simulink model "d_009_classicalGen_nonunidamp"  (Simulink 9.2)
settings: Solver=ode3  StartTime=0.0  StopTime=10.0  FixedStep=1e-4  RelTol=1e-3  EnableMultiTasking=on
libraries: fm_lib x2
settings Model: Creator=fmilano  LastModifiedBy=sl48876  ExtModeAutoUpdateStatusClock=off
settings OptimizationCC: BooleanDataType=off  InitFltsAndDblsToZero=on
settings DebuggingCC: SaveWithParameterizedLinksMsg=none  SignalResolutionControl=TryResolveAllWithWarning  MultiTaskDSMMsg=warning  MultiTaskCondExecSysMsg=none  FcnCallInpInsideContextMsg=error  StateNameClashWarn=none
settings HardwareCC: TargetUnknown=on
settings GRTTargetCC: TargetFcnLib=ansi_tfl_tmw.mat  CodeReplacementLibrary=ANSI_C  CompOptLevelCompliant=off  CPPClassGenCompliant=off
settings ConfigComp: CovSFcnEnable=off

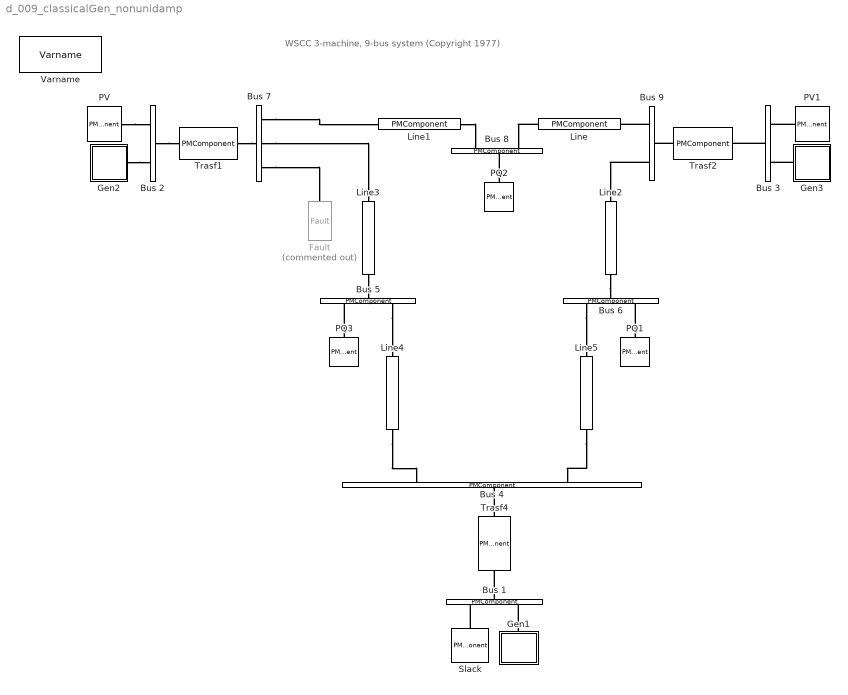
== system d_009_classicalGen_nonunidamp ==
  note: WSCC 3-machine, 9-bus system (Copyright 1977)
  Bus 1 : PMComponent  Tag=PSATblock  Description=Connection  PhysicalDomain=psatdomain  LeftPortType=p1  RightPortType=p1  LConnTagsString=__newl0|__newl1  RConnTagsString=__newr0  mask(Bus){in=2, out=1, p2q=16.5, p3_4q=[1.00   0.00], p5q=4, p6q=1}
      mask prompts: in "Number of inputs:"; out "Number of outputs:"; p2q "Voltage Rating [kV]"; p3_4q "Voltage initial guess [p.u.  rad]"; p5q "Area number"; p6q "Region number"
      mask help: Bus block.
      mask init:
      | fm_inout
      mask Callback p5q: fm_block
      mask Display: plot([0 1 1 0 0],[0 0 1 1 0])
  Bus 2 : PMComponent  Tag=PSATblock  Description=Connection  PhysicalDomain=psatdomain  LeftPortType=p1  RightPortType=p1  LConnTagsString=__newl0|__newl1  RConnTagsString=__newr0  mask(Bus){in=2, out=1, p2q=18, p3_4q=[1.00   0.00], p5q=5, p6q=1}
      mask prompts: in "Number of inputs:"; out "Number of outputs:"; p2q "Voltage Rating [kV]"; p3_4q "Voltage initial guess [p.u.  rad]"; p5q "Area number"; p6q "Region number"
      mask help: Bus block.
      mask init:
      | fm_inout
      mask Callback p5q: fm_block
      mask Display: plot([0 1 1 0 0],[0 0 1 1 0])
  Bus 3 : PMComponent  Tag=PSATblock  Description=Connection  PhysicalDomain=psatdomain  LeftPortType=p1  RightPortType=p1  LConnTagsString=__newl0|__newl1  RConnTagsString=__newr0  mask(Bus){in=2, out=1, p2q=13.8, p3_4q=[1.00   0.00], p5q=3, p6q=1}
      mask prompts: in "Number of inputs:"; out "Number of outputs:"; p2q "Voltage Rating [kV]"; p3_4q "Voltage initial guess [p.u.  rad]"; p5q "Area number"; p6q "Region number"
      mask help: Bus block.
      mask init:
      | fm_inout
      mask Callback p5q: fm_block
      mask Display: plot([0 1 1 0 0],[0 0 1 1 0])
  Bus 4 : PMComponent  Tag=PSATblock  Description=Connection  PhysicalDomain=psatdomain  LeftPortType=p1  RightPortType=p1  LConnTagsString=__newl0|__newl1  RConnTagsString=__newr0  mask(Bus){in=2, out=1, p2q=230, p3_4q=[1.00   0.00], p5q=2, p6q=1}
      mask prompts: in "Number of inputs:"; out "Number of outputs:"; p2q "Voltage Rating [kV]"; p3_4q "Voltage initial guess [p.u.  rad]"; p5q "Area number"; p6q "Region number"
      mask help: Bus block.
      mask init:
      | fm_inout
      mask Callback p5q: fm_block
      mask Display: plot([0 1 1 0 0],[0 0 1 1 0])
  Bus 5 : PMComponent  Tag=PSATblock  Description=Connection  PhysicalDomain=psatdomain  LeftPortType=p1  RightPortType=p1  LConnTagsString=__newl0  RConnTagsString=__newr0|__newr1  mask(Bus){in=1, out=2, p2q=230, p3_4q=[1.00   0.00], p5q=2, p6q=1}
      mask prompts: in "Number of inputs:"; out "Number of outputs:"; p2q "Voltage Rating [kV]"; p3_4q "Voltage initial guess [p.u.  rad]"; p5q "Area number"; p6q "Region number"
      mask help: Bus block.
      mask init:
      | fm_inout
      mask Callback p5q: fm_block
      mask Display: plot([0 1 1 0 0],[0 0 1 1 0])
  Bus 6 : PMComponent  Tag=PSATblock  Description=Connection  PhysicalDomain=psatdomain  LeftPortType=p1  RightPortType=p1  LConnTagsString=__newl0  RConnTagsString=__newr0|__newr1  mask(Bus){in=1, out=2, p2q=230, p3_4q=[1.00   0.00], p5q=2, p6q=1}
      mask prompts: in "Number of inputs:"; out "Number of outputs:"; p2q "Voltage Rating [kV]"; p3_4q "Voltage initial guess [p.u.  rad]"; p5q "Area number"; p6q "Region number"
      mask help: Bus block.
      mask init:
      | fm_inout
      mask Callback p5q: fm_block
      mask Display: plot([0 1 1 0 0],[0 0 1 1 0])
  Bus 7 : PMComponent  Tag=PSATblock  Description=Connection  PhysicalDomain=psatdomain  LeftPortType=p1  RightPortType=p1  LConnTagsString=__newl0  RConnTagsString=__newr0|__newr1|__newr2  mask(Bus){in=1, out=3, p2q=230, p3_4q=[1.00   0.00], p5q=2, p6q=1}
      mask prompts: in "Number of inputs:"; out "Number of outputs:"; p2q "Voltage Rating [kV]"; p3_4q "Voltage initial guess [p.u.  rad]"; p5q "Area number"; p6q "Region number"
      mask help: Bus block.
      mask init:
      | fm_inout
      mask Callback p5q: fm_block
      mask Display: plot([0 1 1 0 0],[0 0 1 1 0])
  Bus 8 : PMComponent  Tag=PSATblock  Description=Connection  PhysicalDomain=psatdomain  LeftPortType=p1  RightPortType=p1  LConnTagsString=__newl0|__newl1  RConnTagsString=__newr0  mask(Bus){in=2, out=1, p2q=230, p3_4q=[1.00   0.00], p5q=2, p6q=1}
      mask prompts: in "Number of inputs:"; out "Number of outputs:"; p2q "Voltage Rating [kV]"; p3_4q "Voltage initial guess [p.u.  rad]"; p5q "Area number"; p6q "Region number"
      mask help: Bus block.
      mask init:
      | fm_inout
      mask Callback p5q: fm_block
      mask Display: plot([0 1 1 0 0],[0 0 1 1 0])
  Bus 9 : PMComponent  Tag=PSATblock  Description=Connection  PhysicalDomain=psatdomain  LeftPortType=p1  RightPortType=p1  LConnTagsString=__newl0  RConnTagsString=__newr0|__newr1  mask(Bus){in=1, out=2, p2q=230, p3_4q=[1.00   0.00], p5q=2, p6q=1}
      mask prompts: in "Number of inputs:"; out "Number of outputs:"; p2q "Voltage Rating [kV]"; p3_4q "Voltage initial guess [p.u.  rad]"; p5q "Area number"; p6q "Region number"
      mask help: Bus block.
      mask init:
      | fm_inout
      mask Callback p5q: fm_block
      mask Display: plot([0 1 1 0 0],[0 0 1 1 0])
  Fault : fm_lib/Faults &  Breakers/Fault  Tag=PSATblock  Description=Faults & Breakers  Commented=on  LConnTagsString=__newl0  p2_3_4q="[100  400  60]"  p5q=1.00  p6q=1.0025  p7q=1e-5  p8q=1e-3
  Gen1 : Subsystem  Tag=PSATblock  Description=Machines  mask(Syn){p2_3_4q=[100  16.5   60], p5q=2, p7_6q=[0.00  0.00], p8_9_10q=[0.1460  0.0608  0.0000], p11_12q=[8.96  0.00], p13_14_15q=[0.0969  0.0969  0.0000], p16_17q=[0.310  0.0000], p18_19q=[2*23.64  0.1*47.28], p20_21q=[0.00  0.00], p22_23q=[1.00  1.00], p24q=0.002, p25_26q=[0 0], in=0, p27q=1, p28q=on}
      mask prompts: p2_3_4q "Power, voltage and frequency ratings [MVA, kV, Hz]"; p5q "Machine Dynamic Order"; p7_6q "resistance ra and leakage reactance xl [p.u. p.u.]"; p8_9_10q "d-axis reactances Xd, X'd X"d [p.u.,p.u.,p.u.]"; p11_12q "d-axis open circuit time constants T'd0 and T"d0 [s, s]"; p13_14_15q "q-axis reactances Xq, X'q, X"q [p.u.  p.u.  p.u.]"; p16_17q "q-axis open circuit time constants T'q0 and T"q0 [s s]"; p18_19q "Inertia (M = 2H) and Damping [s, p.u.]"; p20_21q "Speed and active power additional signals Kw and Kp [p.u., p.u.]"; p22_23q "Percentage of active and reactive powers at bus [p.u. p.u.]"; p24q "d-axis additional circuit leakage time constant Taa [s]"; p25_26q "Saturation coefficients S(1.0) and S(1.2)"; in "Number of input signals"; p27q "COI number"; p28q "Connected"
      mask help: This block defines a fourth order synchronous machine.
      mask init:
      | fm_inout
      | [x,y] = fm_draw('circle');
      | [xg,yg] = fm_draw('G');
      | [xs,ys] = fm_draw('sinus');
      mask TypeOptions p5q: 8 | 6 | 5.3 | 5.2 | 5.1 | 4 | 3 | 2
      mask Callback p5q: fm_block
      mask TypeOptions in: 0 | 1 | 2
      mask Callback p28q: fm_block
      mask Display:
      | plot(x+1.4,y,0.12*xs+1,0.15*ys-0.6)
      | color('blue')
      | plot(1.4+0.45*xg,0.3+0.45*yg)
  Gen2 : Subsystem  Tag=PSATblock  Description=Machines  mask(Syn){p2_3_4q=[100  18   60], p5q=2, p7_6q=[0.00  0.00], p8_9_10q=[0.8958  0.1198  0.0000], p11_12q=[6.00  0.00], p13_14_15q=[0.8645  0.1969  0.0000], p16_17q=[0.5350  0.0000], p18_19q=[12.80  0.2*12.80], p20_21q=[0.00  0.00], p22_23q=[1.00  1.00], p24q=0.002, p25_26q=[0 0], in=0, p27q=1, p28q=on}
      mask prompts: p2_3_4q "Power, voltage and frequency ratings [MVA, kV, Hz]"; p5q "Machine Dynamic Order"; p7_6q "resistance ra and leakage reactance xl [p.u. p.u.]"; p8_9_10q "d-axis reactances Xd, X'd X"d [p.u.,p.u.,p.u.]"; p11_12q "d-axis open circuit time constants T'd0 and T"d0 [s, s]"; p13_14_15q "q-axis reactances Xq, X'q, X"q [p.u.  p.u.  p.u.]"; p16_17q "q-axis open circuit time constants T'q0 and T"q0 [s s]"; p18_19q "Inertia (M = 2H) and Damping [s, p.u.]"; p20_21q "Speed and active power additional signals Kw and Kp [p.u., p.u.]"; p22_23q "Percentage of active and reactive powers at bus [p.u. p.u.]"; p24q "d-axis additional circuit leakage time constant Taa [s]"; p25_26q "Saturation coefficients S(1.0) and S(1.2)"; in "Number of input signals"; p27q "COI number"; p28q "Connected"
      mask help: This block defines a fourth order synchronous machine.
      mask init:
      | fm_inout
      | [x,y] = fm_draw('circle');
      | [xg,yg] = fm_draw('G');
      | [xs,ys] = fm_draw('sinus');
      mask TypeOptions p5q: 8 | 6 | 5.3 | 5.2 | 5.1 | 4 | 3 | 2
      mask Callback p5q: fm_block
      mask TypeOptions in: 0 | 1 | 2
      mask Callback p28q: fm_block
      mask Display:
      | plot(x+1.4,y,0.12*xs+1,0.15*ys-0.6)
      | color('blue')
      | plot(1.4+0.45*xg,0.3+0.45*yg)
  Gen3 : Subsystem  Tag=PSATblock  Description=Machines  mask(Syn){p2_3_4q=[100  13.8   60], p5q=2, p7_6q=[0.00  0.00], p8_9_10q=[1.3125  0.1813  0.0000], p11_12q=[5.89  0.00], p13_14_15q=[1.2578  0.2500  0.0000], p16_17q=[0.600  0.0000], p18_19q=[6.02  0.3*6.02], p20_21q=[0.00  0.00], p22_23q=[1.00  1.00], p24q=0.002, p25_26q=[0 0], in=0, p27q=1, p28q=on}
      mask prompts: p2_3_4q "Power, voltage and frequency ratings [MVA, kV, Hz]"; p5q "Machine Dynamic Order"; p7_6q "resistance ra and leakage reactance xl [p.u. p.u.]"; p8_9_10q "d-axis reactances Xd, X'd X"d [p.u.,p.u.,p.u.]"; p11_12q "d-axis open circuit time constants T'd0 and T"d0 [s, s]"; p13_14_15q "q-axis reactances Xq, X'q, X"q [p.u.  p.u.  p.u.]"; p16_17q "q-axis open circuit time constants T'q0 and T"q0 [s s]"; p18_19q "Inertia (M = 2H) and Damping [s, p.u.]"; p20_21q "Speed and active power additional signals Kw and Kp [p.u., p.u.]"; p22_23q "Percentage of active and reactive powers at bus [p.u. p.u.]"; p24q "d-axis additional circuit leakage time constant Taa [s]"; p25_26q "Saturation coefficients S(1.0) and S(1.2)"; in "Number of input signals"; p27q "COI number"; p28q "Connected"
      mask help: This block defines a fourth order synchronous machine.
      mask init:
      | fm_inout
      | [x,y] = fm_draw('circle');
      | [xg,yg] = fm_draw('G');
      | [xs,ys] = fm_draw('sinus');
      mask TypeOptions p5q: 8 | 6 | 5.3 | 5.2 | 5.1 | 4 | 3 | 2
      mask Callback p5q: fm_block
      mask TypeOptions in: 0 | 1 | 2
      mask Callback p28q: fm_block
      mask Display:
      | plot(x+1.4,y,0.12*xs+1,0.15*ys-0.6)
      | color('blue')
      | plot(1.4+0.45*xg,0.3+0.45*yg)
  Line : PMComponent  Tag=PSATblock  Description=Power Flow  PhysicalDomain=psatdomain  LeftPortType=p1  RightPortType=p1  LConnTagsString=__newl0  RConnTagsString=__newr0  mask(Line){p3_4_5q=[100  230  60], p6q=0, p8q=0.0119, p9q=0.1008, p10q=0.1045*2, p13_14_15q=[0.0  0.0  0.0], p16q=on}
      mask prompts: p3_4_5q "Power, Voltage and Frequency Ratings [MVA, kV, Hz]"; p6q "Length of line [km] (0 for p.u. parameters)"; p8q "Resistance [p.u. (Ohms/km)]"; p9q "Reactance [p.u. (H/km)]"; p10q "Susceptance [p.u. (F/km)]"; p13_14_15q "Imax, Pmax and Smax [p.u., p.u., p.u.]"; p16q "Connected"
      mask help: This block defines a pi model for a tree phase line.
      mask init:
      | [xp,yp] = fm_draw('pi');
      mask Callback p16q: fm_block
      mask Display:
      | plot([-1  1  1 -1 -1],[-0.2 -0.2 0.2 0.2 -0.2])
      | color('blue')
      | plot(0.35*xp,0.2*yp)
  Line1 : PMComponent  Tag=PSATblock  Description=Power Flow  PhysicalDomain=psatdomain  LeftPortType=p1  RightPortType=p1  LConnTagsString=__newl0  RConnTagsString=__newr0  mask(Line){p3_4_5q=[100  230  60], p6q=0, p8q=0.0085, p9q=0.072*5, p10q=0.0745*2, p13_14_15q=[0.0  0.0  0.0], p16q=on}
      mask prompts: p3_4_5q "Power, Voltage and Frequency Ratings [MVA, kV, Hz]"; p6q "Length of line [km] (0 for p.u. parameters)"; p8q "Resistance [p.u. (Ohms/km)]"; p9q "Reactance [p.u. (H/km)]"; p10q "Susceptance [p.u. (F/km)]"; p13_14_15q "Imax, Pmax and Smax [p.u., p.u., p.u.]"; p16q "Connected"
      mask help: This block defines a pi model for a tree phase line.
      mask init:
      | [xp,yp] = fm_draw('pi');
      mask Callback p16q: fm_block
      mask Display:
      | plot([-1  1  1 -1 -1],[-0.2 -0.2 0.2 0.2 -0.2])
      | color('blue')
      | plot(0.35*xp,0.2*yp)
  Line2 : PMComponent  Tag=PSATblock  Description=Power Flow  PhysicalDomain=psatdomain  LeftPortType=p1  RightPortType=p1  LConnTagsString=__newl0  RConnTagsString=__newr0  mask(Line){p3_4_5q=[100  230  60], p6q=0, p8q=0.039, p9q=0.170*5, p10q=0.179*2, p13_14_15q=[0.0  0.0  0.0], p16q=on}
      mask prompts: p3_4_5q "Power, Voltage and Frequency Ratings [MVA, kV, Hz]"; p6q "Length of line [km] (0 for p.u. parameters)"; p8q "Resistance [p.u. (Ohms/km)]"; p9q "Reactance [p.u. (H/km)]"; p10q "Susceptance [p.u. (F/km)]"; p13_14_15q "Imax, Pmax and Smax [p.u., p.u., p.u.]"; p16q "Connected"
      mask help: This block defines a pi model for a tree phase line.
      mask init:
      | [xp,yp] = fm_draw('pi');
      mask Callback p16q: fm_block
      mask Display:
      | plot([-1  1  1 -1 -1],[-0.2 -0.2 0.2 0.2 -0.2])
      | color('blue')
      | plot(0.35*xp,0.2*yp)
  Line3 : PMComponent  Tag=PSATblock  Description=Power Flow  PhysicalDomain=psatdomain  LeftPortType=p1  RightPortType=p1  LConnTagsString=__newl0  RConnTagsString=__newr0  mask(Line){p3_4_5q=[100  230  60], p6q=0, p8q=0.032, p9q=0.161*5, p10q=0.153*2, p13_14_15q=[0.0  0.0  0.0], p16q=on}
      mask prompts: p3_4_5q "Power, Voltage and Frequency Ratings [MVA, kV, Hz]"; p6q "Length of line [km] (0 for p.u. parameters)"; p8q "Resistance [p.u. (Ohms/km)]"; p9q "Reactance [p.u. (H/km)]"; p10q "Susceptance [p.u. (F/km)]"; p13_14_15q "Imax, Pmax and Smax [p.u., p.u., p.u.]"; p16q "Connected"
      mask help: This block defines a pi model for a tree phase line.
      mask init:
      | [xp,yp] = fm_draw('pi');
      mask Callback p16q: fm_block
      mask Display:
      | plot([-1  1  1 -1 -1],[-0.2 -0.2 0.2 0.2 -0.2])
      | color('blue')
      | plot(0.35*xp,0.2*yp)
  Line4 : PMComponent  Tag=PSATblock  Description=Power Flow  PhysicalDomain=psatdomain  LeftPortType=p1  RightPortType=p1  LConnTagsString=__newl0  RConnTagsString=__newr0  mask(Line){p3_4_5q=[100  230  60], p6q=0, p8q=0.01, p9q=0.085, p10q=0.088*2, p13_14_15q=[0.0  0.0  0.0], p16q=on}
      mask prompts: p3_4_5q "Power, Voltage and Frequency Ratings [MVA, kV, Hz]"; p6q "Length of line [km] (0 for p.u. parameters)"; p8q "Resistance [p.u. (Ohms/km)]"; p9q "Reactance [p.u. (H/km)]"; p10q "Susceptance [p.u. (F/km)]"; p13_14_15q "Imax, Pmax and Smax [p.u., p.u., p.u.]"; p16q "Connected"
      mask help: This block defines a pi model for a tree phase line.
      mask init:
      | [xp,yp] = fm_draw('pi');
      mask Callback p16q: fm_block
      mask Display:
      | plot([-1  1  1 -1 -1],[-0.2 -0.2 0.2 0.2 -0.2])
      | color('blue')
      | plot(0.35*xp,0.2*yp)
  Line5 : PMComponent  Tag=PSATblock  Description=Power Flow  PhysicalDomain=psatdomain  LeftPortType=p1  RightPortType=p1  LConnTagsString=__newl0  RConnTagsString=__newr0  mask(Line){p3_4_5q=[100  230  60], p6q=0, p8q=0.017, p9q=0.092, p10q=0.079*2, p13_14_15q=[0.0  0.0  0.0], p16q=on}
      mask prompts: p3_4_5q "Power, Voltage and Frequency Ratings [MVA, kV, Hz]"; p6q "Length of line [km] (0 for p.u. parameters)"; p8q "Resistance [p.u. (Ohms/km)]"; p9q "Reactance [p.u. (H/km)]"; p10q "Susceptance [p.u. (F/km)]"; p13_14_15q "Imax, Pmax and Smax [p.u., p.u., p.u.]"; p16q "Connected"
      mask help: This block defines a pi model for a tree phase line.
      mask init:
      | [xp,yp] = fm_draw('pi');
      mask Callback p16q: fm_block
      mask Display:
      | plot([-1  1  1 -1 -1],[-0.2 -0.2 0.2 0.2 -0.2])
      | color('blue')
      | plot(0.35*xp,0.2*yp)
  PQ1 : PMComponent  Tag=PSATblock  Description=Power Flow  PhysicalDomain=psatdomain  LeftPortType=p1  RightPortType=p1  LConnTagsString=__newl0  mask(PQ){p2_3q=[100  230], p4_5q=[0.90  0.30], p6_7q=[1.2  0.8], p8q=off, p9q=on}
      mask prompts: p2_3q "Power and Voltage Ratings [MVA, kV]"; p4_5q "Active and Reactive Powers [p.u.  p.u.]"; p6_7q "Maximum and Minimum Allowable Voltage [p.u.   p.u.]"; p8q "Allow conversion to impendance for min & max voltage"; p9q "Connected"
      mask help:
      | This block defines a constant power load:
      |
      | P = Pcost.
      | Q = Qcost.
      mask Callback p8q: fm_block
      mask Callback p9q: fm_block
      mask Display: plot([1 -0.5 -0.5 1],[0 0.866 -0.866 0])
  PQ2 : PMComponent  Tag=PSATblock  Description=Power Flow  PhysicalDomain=psatdomain  LeftPortType=p1  RightPortType=p1  LConnTagsString=__newl0  mask(PQ){p2_3q=[100  230], p4_5q=[1.00  0.35], p6_7q=[1.2  0.8], p8q=off, p9q=on}
      mask prompts: p2_3q "Power and Voltage Ratings [MVA, kV]"; p4_5q "Active and Reactive Powers [p.u.  p.u.]"; p6_7q "Maximum and Minimum Allowable Voltage [p.u.   p.u.]"; p8q "Allow conversion to impendance for min & max voltage"; p9q "Connected"
      mask help:
      | This block defines a constant power load:
      |
      | P = Pcost.
      | Q = Qcost.
      mask Callback p8q: fm_block
      mask Callback p9q: fm_block
      mask Display: plot([1 -0.5 -0.5 1],[0 0.866 -0.866 0])
  PQ3 : PMComponent  Tag=PSATblock  Description=Power Flow  PhysicalDomain=psatdomain  LeftPortType=p1  RightPortType=p1  LConnTagsString=__newl0  mask(PQ){p2_3q=[100  230], p4_5q=[1.25  0.50], p6_7q=[1.2  0.8], p8q=off, p9q=on}
      mask prompts: p2_3q "Power and Voltage Ratings [MVA, kV]"; p4_5q "Active and Reactive Powers [p.u.  p.u.]"; p6_7q "Maximum and Minimum Allowable Voltage [p.u.   p.u.]"; p8q "Allow conversion to impendance for min & max voltage"; p9q "Connected"
      mask help:
      | This block defines a constant power load:
      |
      | P = Pcost.
      | Q = Qcost.
      mask Callback p8q: fm_block
      mask Callback p9q: fm_block
      mask Display: plot([1 -0.5 -0.5 1],[0 0.866 -0.866 0])
  PV : PMComponent  Tag=PSATblock  Description=Power Flow  PhysicalDomain=psatdomain  LeftPortType=p1  RightPortType=p1  RConnTagsString=__newr0  mask(PV){p2_3q=[100  18], p4q=1.63, p5q=1.025, p6_7q=[99 -99], p8_9q=[1.1  0.9], p10q=1, p11q=on}
      mask prompts: p2_3q "Power and Voltage Ratings [MVA, kV]"; p4q "Active Power [p.u.]"; p5q "Voltage Magnitude [p.u.]"; p6_7q "Qmax and Qmin [p.u.  p.u.]"; p8_9q "Vmax and Vmin [p.u.  p.u.]"; p10q "Loss Participation Factor"; p11q "Connected"
      mask help:
      | This block defines a PV bus for load flow studies:
      |
      | P = Pcost.
      | V = Vdes.
      mask init:
      | [x,y] = fm_draw('circle');
      | [xp,yp] = fm_draw('P');
      mask Callback p11q: fm_block
      mask Display:
      | plot(x,y)
      | color('blue')
      | plot(0.3*xp-0.35,0.6*yp,[0.1 0.3 0.5],[0.3 -0.3 0.3])
  PV1 : PMComponent  Tag=PSATblock  Description=Power Flow  PhysicalDomain=psatdomain  LeftPortType=p1  RightPortType=p1  RConnTagsString=__newr0  mask(PV){p2_3q=[100  13.8], p4q=0.85, p5q=1.025, p6_7q=[99  -99], p8_9q=[1.1  0.9], p10q=1, p11q=on}
      mask prompts: p2_3q "Power and Voltage Ratings [MVA, kV]"; p4q "Active Power [p.u.]"; p5q "Voltage Magnitude [p.u.]"; p6_7q "Qmax and Qmin [p.u.  p.u.]"; p8_9q "Vmax and Vmin [p.u.  p.u.]"; p10q "Loss Participation Factor"; p11q "Connected"
      mask help:
      | This block defines a PV bus for load flow studies:
      |
      | P = Pcost.
      | V = Vdes.
      mask init:
      | [x,y] = fm_draw('circle');
      | [xp,yp] = fm_draw('P');
      mask Callback p11q: fm_block
      mask Display:
      | plot(x,y)
      | color('blue')
      | plot(0.3*xp-0.35,0.6*yp,[0.1 0.3 0.5],[0.3 -0.3 0.3])
  Slack : PMComponent  Tag=PSATblock  Description=Power Flow  PhysicalDomain=psatdomain  LeftPortType=p1  RightPortType=p1  RConnTagsString=__newr0  mask(SW){p2_3q=[100  16.5], p4q=1.04, p5q=0.00, p6_7q=[99 -99], p8_9q=[1.1  0.9], p10q=0.80, p11q=1, p12q=on, p13q=on}
      mask prompts: p2_3q "Power and Voltage Ratings [MVA, kV]"; p4q "Voltage Magnitude [p.u.]"; p5q "Reference Phase Angle [rad]"; p6_7q "Qmax and Qmin [p.u.  p.u.]"; p8_9q "Vmax and Vmin  [p.u.  p.u.]"; p10q "Active Power Guess [p.u.]"; p11q "Loss Participation Factor"; p12q "Reference bus"; p13q "Connected"
      mask help:
      | This block defines a V-theta bus:
      |
      | V = V_des
      | theta = theta_des
      mask init:
      | [x,y] = fm_draw('circle');
      | [xt,yt] = fm_draw('theta');
      mask Callback p12q: fm_block
      mask Callback p13q: fm_block
      mask Display: plot([0 1 1 0 0],[0 0 1 1 0]), color('blue'), plot([0 1],[0 1],[0 1],[1 0],[0.5 1 0.5 0 0.5],[0 0.5 1 0.5 0])
  Trasf1 : PMComponent  Tag=PSATblock  Description=Power Flow  PhysicalDomain=psatdomain  LeftPortType=p1  RightPortType=p1  LConnTagsString=__newl0  RConnTagsString=__newr0  mask(Line){p3_4_5q=[100  18  60], p7q=18/230, p8q=0.0, p9q=0.0625, p13_14_15q=[0.0  0.0  0.0], p16q=on}
      mask prompts: p3_4_5q "Power, Voltage and Frequency Ratings [MVA, kV, Hz]"; p7q "Primary and secondary voltage ratio [kV/kV]"; p8q "Resistance [p.u.]"; p9q "Reactance [p.u.]"; p13_14_15q "Imax, Pmax and Smax [p.u., p.u., p.u.]"; p16q "Connected"
      mask help: This block defines a transformer.
      mask init:
      | [x,y] = fm_draw('circle');
      | [x1,y1] = fm_draw('1');
      | [x2,y2] = fm_draw('2');
      mask Callback p16q: fm_block
      mask Display:
      | plot(x,y,x+1.4,y,[-1 -1.3],[0 0],[2.4 2.7],[0 0])
      | color('green')
      | plot(-0.1+0.65*x1,0.65*y1)
      | plot(1.5+0.65*x2,0.65*y2)
  Trasf2 : PMComponent  Tag=PSATblock  Description=Power Flow  PhysicalDomain=psatdomain  LeftPortType=p1  RightPortType=p1  LConnTagsString=__newl0  RConnTagsString=__newr0  mask(Line){p3_4_5q=[100  13.8  60], p7q=13.8/230, p8q=0.0, p9q=0.0586, p13_14_15q=[0.0  0.0  0.0], p16q=on}
      mask prompts: p3_4_5q "Power, Voltage and Frequency Ratings [MVA, kV, Hz]"; p7q "Primary and secondary voltage ratio [kV/kV]"; p8q "Resistance [p.u.]"; p9q "Reactance [p.u.]"; p13_14_15q "Imax, Pmax and Smax [p.u., p.u., p.u.]"; p16q "Connected"
      mask help: This block defines a transformer.
      mask init:
      | [x,y] = fm_draw('circle');
      | [x1,y1] = fm_draw('1');
      | [x2,y2] = fm_draw('2');
      mask Callback p16q: fm_block
      mask Display:
      | plot(x,y,x+1.4,y,[-1 -1.3],[0 0],[2.4 2.7],[0 0])
      | color('green')
      | plot(-0.1+0.65*x1,0.65*y1)
      | plot(1.5+0.65*x2,0.65*y2)
  Trasf4 : PMComponent  Tag=PSATblock  Description=Power Flow  PhysicalDomain=psatdomain  LeftPortType=p1  RightPortType=p1  LConnTagsString=__newl0  RConnTagsString=__newr0  mask(Line){p3_4_5q=[100  16.5  60], p7q=16.5/230, p8q=0.0, p9q=0.0576, p13_14_15q=[0.0  0.0  0.0], p16q=on}
      mask prompts: p3_4_5q "Power, Voltage and Frequency Ratings [MVA, kV, Hz]"; p7q "Primary and secondary voltage ratio [kV/kV]"; p8q "Resistance [p.u.]"; p9q "Reactance [p.u.]"; p13_14_15q "Imax, Pmax and Smax [p.u., p.u., p.u.]"; p16q "Connected"
      mask help: This block defines a transformer.
      mask init:
      | [x,y] = fm_draw('circle');
      | [x1,y1] = fm_draw('1');
      | [x2,y2] = fm_draw('2');
      mask Callback p16q: fm_block
      mask Display:
      | plot(x,y,x+1.4,y,[-1 -1.3],[0 0],[2.4 2.7],[0 0])
      | color('green')
      | plot(-0.1+0.65*x1,0.65*y1)
      | plot(1.5+0.65*x2,0.65*y2)
  Varname : fm_lib/Connections/Varname  Tag=PSATblock  Description=OPF & CPF  pxq="[1  2  3  4  5  6  7  8  9  10  11  12  13  14  15  16  17  18  19  20  21  22  23  24  25  26  27  28  29  30  31  32  33  34  35  36  37  38  39  40  41  42  43  44  45  55  56  57  58  59  60  61  62  63  64  65  66  67  68  69  70  71  72]"
  connections:
  Bus 7/RConn2 -- Line3/LConn1
  Gen3/RConn1 -- Bus 3/LConn2
  Gen2/RConn1 -- Bus 2/LConn2
  Line5/RConn1 -- Bus 4/LConn2
  Line4/RConn1 -- Bus 4/LConn1
  Bus 5/RConn2 -- Line4/LConn1
  Bus 6/RConn1 -- Line5/LConn1
  Line3/RConn1 -- Bus 5/LConn1
  Line2/RConn1 -- Bus 6/LConn1
  Bus 9/RConn2 -- Line2/LConn1
  Line/RConn1 -- Bus 8/LConn2
  Bus 7/RConn1 -- Line1/LConn1
  Bus 9/RConn1 -- Line/LConn1
  Trasf2/RConn1 -- Bus 9/LConn1
  Trasf1/RConn1 -- Bus 7/LConn1
  Bus 3/RConn1 -- Trasf2/LConn1
  Bus 2/RConn1 -- Trasf1/LConn1
  PV1/RConn1 -- Bus 3/LConn1
  PV/RConn1 -- Bus 2/LConn1
  PQ1/LConn1 -- Bus 6/RConn2
  PQ2/LConn1 -- Bus 8/RConn1
  PQ3/LConn1 -- Bus 5/RConn1
  Line1/RConn1 -- Bus 8/LConn1
  Trasf4/RConn1 -- Bus 4/RConn1
  Bus 1/RConn1 -- Trasf4/LConn1
  Slack/RConn1 -- Bus 1/LConn1
  Gen1/RConn1 -- Bus 1/LConn2
  Bus 7/RConn3 -- Fault/LConn1

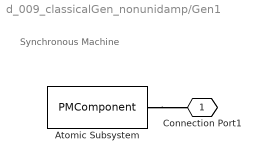
== system d_009_classicalGen_nonunidamp/Gen1 ==
  note: Synchronous Machine
  Atomic Subsystem : PMComponent  PhysicalDomain=psatdomain  LeftPortType=p1  RightPortType=p1  RConnTagsString=__newr0
  Connection Port1 : PMIOPort  Tag=PMCPort  Side=Right
  connections:
  Atomic Subsystem/RConn1 -- Connection Port1/RConn1

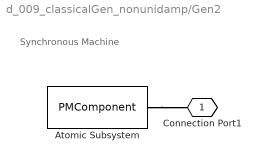
== system d_009_classicalGen_nonunidamp/Gen2 ==
  note: Synchronous Machine
  Atomic Subsystem : PMComponent  PhysicalDomain=psatdomain  LeftPortType=p1  RightPortType=p1  RConnTagsString=__newr0
  Connection Port1 : PMIOPort  Tag=PMCPort  Side=Right
  connections:
  Atomic Subsystem/RConn1 -- Connection Port1/RConn1

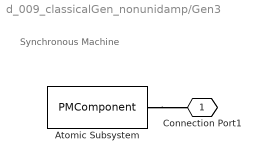
== system d_009_classicalGen_nonunidamp/Gen3 ==
  note: Synchronous Machine
  Atomic Subsystem : PMComponent  PhysicalDomain=psatdomain  LeftPortType=p1  RightPortType=p1  RConnTagsString=__newr0
  Connection Port1 : PMIOPort  Tag=PMCPort  Side=Right
  connections:
  Atomic Subsystem/RConn1 -- Connection Port1/RConn1
